simulink model "Villasenor22210431"  (R2023a)
settings: Solver=ode15s  StartTime=0.0  StopTime=10.0  MaxStep=1E-3  RelTol=1e-3
libraries: slpidlib x1
settings Model: LastModifiedBy=diegt
settings DataIOCC: ReturnWorkspaceOutputs=off  TimeSaveName=t
settings DebuggingCC: AlgebraicLoopMsg=none  ArtificialAlgebraicLoopMsg=none  MaxConsecutiveZCsMsg=none  ModelReferenceExtraNoncontSigs=none  OperatingPointInterfaceChecksumMismatchMsg=none
settings RTWCC: GPUComputeCapability=5.0

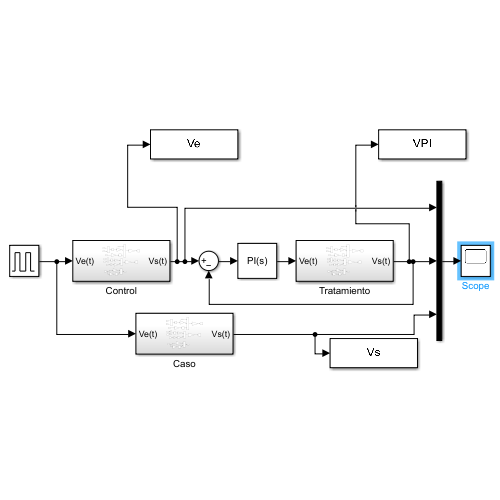
[thumbnail: Simulink's stored preview of the top-level diagram]
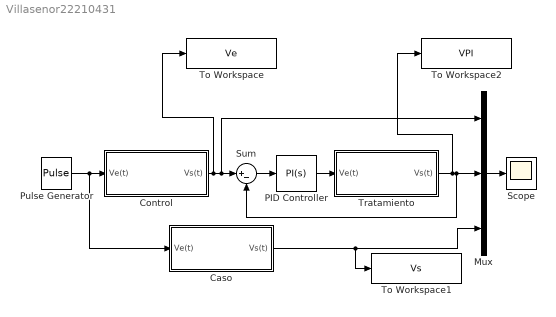
== system Villasenor22210431 ==
  Caso : Subsystem
  Control : Subsystem
  Mux : Mux  Inputs=3
  PID Controller : slpidlib/PID Controller  Controller=PI  Form=Parallel  TimeDomain=Continuous-time  UseExternalTs=off  SampleTime=-1  IntegratorMethod=Forward Euler  FilterMethod=Forward Euler  ControllerParametersSource=internal  P=17.4301980418149  I=212.064703705024  UseKiTs=off  D=0.090937636957781  N=83.1785670178724  UseFilter=on  TunerSelectOption=Transfer Function Based (PID Tuner App)  InitialConditionSource=internal  InitialConditionForIntegrator=0  InitialConditionForFilter=0  DifferentiatorICPrevScaledInput=0  ExternalReset=none  TrackingMode=off  Kt=1  LimitOutput=off  SatLimitsSource=internal  UpperSaturationLimit=inf  LowerSaturationLimit=-inf  LinearizeAsGain=on  AntiWindupMode=none  Kb=1  LimitIntegrator=off  UpperIntegratorSaturationLimit=inf  LowerIntegratorSaturationLimit=-inf  POutMin=[]  POutMax=[]  IOutMin=[]  IOutMax=[]  DOutMin=[]  DOutMax=[]  NOutMin=[]  NOutMax=[]  SumOutMin=[]  SumOutMax=[]  SaturationOutMin=[]  SaturationOutMax=[]  PParamMin=[]  PParamMax=[]  IParamMin=[]  IParamMax=[]  DParamMin=[]  DParamMax=[]  NParamMin=[]  NParamMax=[]  KbParamMin=[]  KbParamMax=[]  KtParamMin=[]  KtParamMax=[]  KbOutMin=[]  KbOutMax=[]  KtOutMin=[]  KtOutMax=[]  IntegratorOutMin=[]  IntegratorOutMax=[]  FilterOutMin=[]  FilterOutMax=[]  SumI1OutMin=[]  SumI1OutMax=[]  SumI2OutMin=[]  SumI2OutMax=[]  SumI3OutMin=[]  SumI3OutMax=[]  SumI4OutMin=[]  SumI4OutMax=[]  SumDOutMin=[]  SumDOutMax=[]  DifferentiatorOutMin=[]  DifferentiatorOutMax=[]  FilterDiffOutCoefMin=[]  FilterDiffOutCoefMax=[]  ReciprocalOutMin=[]  ReciprocalOutMax=[]  SumDenOutMin=[]  SumDenOutMax=[]  SumNumOutMin=[]  SumNumOutMax=[]  DivideOutMin=[]  DivideOutMax=[]  UdiffTsProdOutMin=[]  UdiffTsProdOutMax=[]  NTsProdOutMin=[]  NTsProdOutMax=[]  UintegralTsProdOutMin=[]  UintegralTsProdOutMax=[]  UngainTsProdOutMin=[]  UngainTsProdOutMax=[]  ClampingZeroOutDataTypeStr=Inherit: Inherit via back propagation  ClampingZeroOutMin=[]  ClampingZeroOutMax=[]  FilterDenConstantOutDataTypeStr=Inherit: Inherit via back propagation  FilterDenConstantOutMin=[]  FilterDenConstantOutMax=[]  PCopyOutDataTypeStr=Inherit: Inherit via back propagation  PCopyOutMin=[]  PCopyOutMax=[]  NCopyOutDataTypeStr=Inherit: Inherit via back propagation  NCopyOutMin=[]  NCopyOutMax=[]  IntegratorContinuousStateAttributes=''  IntegratorStateMustResolveToSignalObject=off  IntegratorRTWStateStorageClass=Auto  FilterContinuousStateAttributes=''  FilterStateMustResolveToSignalObject=off  FilterRTWStateStorageClass=Auto  ParallelPVariant=InternalParameters  IdealPVariant=Disabled  IVariant=InternalParameters  DVariant=Disabled  IntegratorVariant=Continuous  SatVariant=Disabled  AWVariant=Passthrough  PCopyVariant=Disabled  TRVariant=Disabled  FdbkBlocksVariant=Forward  IdealPFdbkVariant=Disabled  SatFdbkVariant=Disabled  DerivativeFilterVariant=Disabled  NVariant=Disabled  NCopyVariant=Disabled_SignalSpec  FilterICVariant=Disabled  IntegratorICVariant=InternalICs  ExternalResetVariant=Disabled  TRSumVariant=Passthrough  SumFdbkVariant=Disabled  SumVariant=Sum_PI  TsampFilterVariant=InternalTs  TsampNgainVariant=Passthrough  TsampIntegralVariant=Disabled_SignalSpec  ExternalSaturationOutDataTypeStr=Inherit: Same as second input
  Pulse Generator : DiscretePulseGenerator  PulseType=Time based  Period=10  PulseWidth=10  PhaseDelay=1
  Scope : Scope
  Sum : Sum  Inputs=|+-
  To Workspace : ToWorkspace  VariableName=Ve  SampleTime=-1
  To Workspace1 : ToWorkspace  VariableName=Vs  SampleTime=-1
  To Workspace2 : ToWorkspace  VariableName=VPI  SampleTime=-1
  Tratamiento : Subsystem
  wires:
  Mux/1 -> Scope/1
  Sum/1 -> PID Controller/1
  Pulse Generator/1 -> Caso/1(Ve(t)), Control/1(Ve(t))
  Control/1(Vs(t)) -> To Workspace/1, Mux/1, Sum/1
  Caso/1(Vs(t)) -> Mux/3, To Workspace1/1
  PID Controller/1 -> Tratamiento/1(Ve(t))
  Tratamiento/1(Vs(t)) -> Mux/2, Sum/2, To Workspace2/1

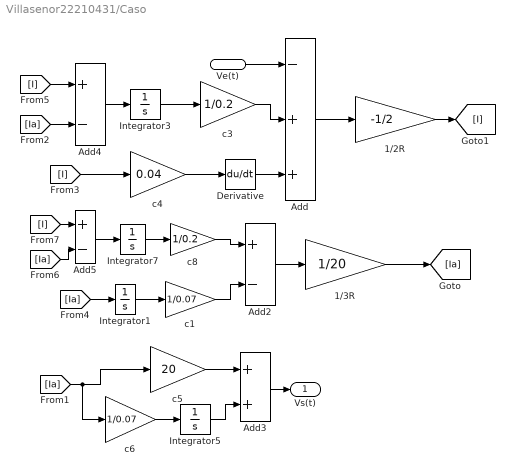
== system Villasenor22210431/Caso ==
  Ve(t) : Inport
  1/2R : Gain  Gain=-1/2
  1/3R : Gain  Gain=1/20
  Add : Sum  Inputs=-++
  Add2 : Sum  Inputs=+-
  Add3 : Sum
  Add4 : Sum  Inputs=+-
  Add5 : Sum  Inputs=+-
  Derivative : Derivative
  Integrator{1,3,5,7} (4 alike) : Integrator
  c1 : Gain  Gain=1/0.07
  c3 : Gain  Gain=1/0.2
  c4 : Gain  Gain=0.04
  c5 : Gain  Gain=20
  c6 : Gain  Gain=1/0.07
  c8 : Gain  Gain=1/0.2
  Vs(t) : Outport
  wires:
  Add2/1 -> 1/3R/1
  Add3/1 -> Vs(t)/1
  Ve(t)/1 -> Add/1
  1/2R/1 -> [I]
  1/3R/1 -> [Ia]
  Integrator3/1 -> c3/1
  c4/1 -> Derivative/1
  c5/1 -> Add3/1
  c6/1 -> Integrator5/1
  Integrator5/1 -> Add3/2
  [Ia] -> c5/1, c6/1
  Add/1 -> 1/2R/1
  c3/1 -> Add/2
  [I] -> c4/1
  Integrator7/1 -> c8/1
  [Ia] -> Integrator1/1
  Integrator1/1 -> c1/1
  [I] -> Add4/1
  [Ia] -> Add4/2
  Add4/1 -> Integrator3/1
  Derivative/1 -> Add/3
  [I] -> Add5/1
  [Ia] -> Add5/2
  Add5/1 -> Integrator7/1
  c1/1 -> Add2/2
  c8/1 -> Add2/1

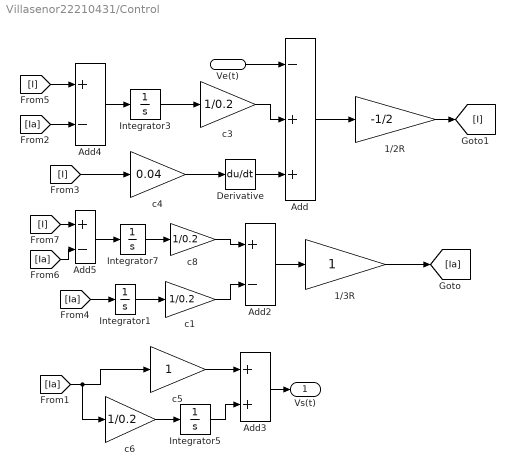
== system Villasenor22210431/Control ==
  Ve(t) : Inport
  1/2R : Gain  Gain=-1/2
  1/3R : Gain
  Add : Sum  Inputs=-++
  Add2 : Sum  Inputs=+-
  Add3 : Sum
  Add4 : Sum  Inputs=+-
  Add5 : Sum  Inputs=+-
  Derivative : Derivative
  Integrator{1,3,5,7} (4 alike) : Integrator
  c{1,3,6,8} (4 alike) : Gain  Gain=1/0.2
  c4 : Gain  Gain=0.04
  c5 : Gain
  Vs(t) : Outport
  wires:
  Add2/1 -> 1/3R/1
  Add3/1 -> Vs(t)/1
  Ve(t)/1 -> Add/1
  1/2R/1 -> [I]
  1/3R/1 -> [Ia]
  Integrator3/1 -> c3/1
  c4/1 -> Derivative/1
  c5/1 -> Add3/1
  c6/1 -> Integrator5/1
  Integrator5/1 -> Add3/2
  [Ia] -> c5/1, c6/1
  Add/1 -> 1/2R/1
  c3/1 -> Add/2
  [I] -> c4/1
  Integrator7/1 -> c8/1
  [Ia] -> Integrator1/1
  Integrator1/1 -> c1/1
  [I] -> Add4/1
  [Ia] -> Add4/2
  Add4/1 -> Integrator3/1
  Derivative/1 -> Add/3
  [I] -> Add5/1
  [Ia] -> Add5/2
  Add5/1 -> Integrator7/1
  c1/1 -> Add2/2
  c8/1 -> Add2/1

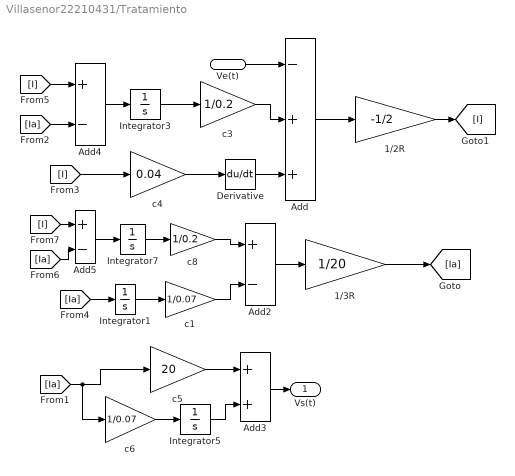
== system Villasenor22210431/Tratamiento ==
  Ve(t) : Inport
  1/2R : Gain  Gain=-1/2
  1/3R : Gain  Gain=1/20
  Add : Sum  Inputs=-++
  Add2 : Sum  Inputs=+-
  Add3 : Sum
  Add4 : Sum  Inputs=+-
  Add5 : Sum  Inputs=+-
  Derivative : Derivative
  Integrator{1,3,5,7} (4 alike) : Integrator
  c1 : Gain  Gain=1/0.07
  c3 : Gain  Gain=1/0.2
  c4 : Gain  Gain=0.04
  c5 : Gain  Gain=20
  c6 : Gain  Gain=1/0.07
  c8 : Gain  Gain=1/0.2
  Vs(t) : Outport
  wires:
  Add2/1 -> 1/3R/1
  Add3/1 -> Vs(t)/1
  Ve(t)/1 -> Add/1
  1/2R/1 -> [I]
  1/3R/1 -> [Ia]
  Integrator3/1 -> c3/1
  c4/1 -> Derivative/1
  c5/1 -> Add3/1
  c6/1 -> Integrator5/1
  Integrator5/1 -> Add3/2
  [Ia] -> c5/1, c6/1
  Add/1 -> 1/2R/1
  c3/1 -> Add/2
  [I] -> c4/1
  Integrator7/1 -> c8/1
  [Ia] -> Integrator1/1
  Integrator1/1 -> c1/1
  [I] -> Add4/1
  [Ia] -> Add4/2
  Add4/1 -> Integrator3/1
  Derivative/1 -> Add/3
  [I] -> Add5/1
  [Ia] -> Add5/2
  Add5/1 -> Integrator7/1
  c1/1 -> Add2/2
  c8/1 -> Add2/1
